simulink model "EquationsOfMotion_EOM"  (R2024b)
settings: Solver=VariableStepAuto  StartTime=0.0  StopTime=10.0  RelTol=1e-3
values from neighbouring files (symbols this model uses):
  g = 9.81    [ParameterInSI.m]    (also in start.m = 9.807)
undefined symbols (not defined in the file or in its folder): ft, INI, m, s
libraries: aerolibconvert2 x3, shared6dof x1, aerolibasang x1, aerolibanimutils x1
settings Model: Creator=the-main  LastModifiedBy=the-main

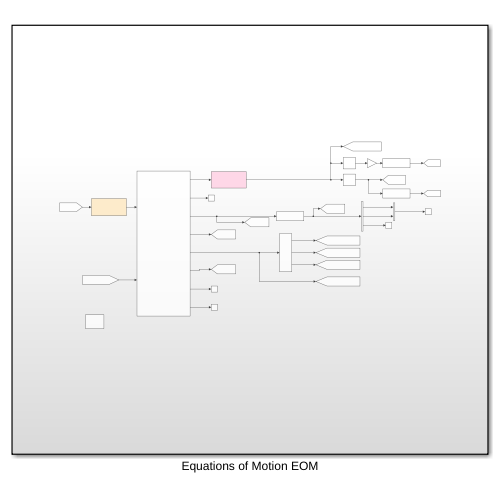
[thumbnail: Simulink's stored preview of the top-level diagram]
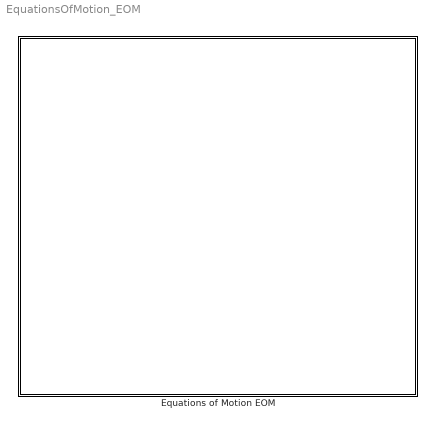
== system EquationsOfMotion_EOM ==
  Equations of Motion EOM : Subsystem

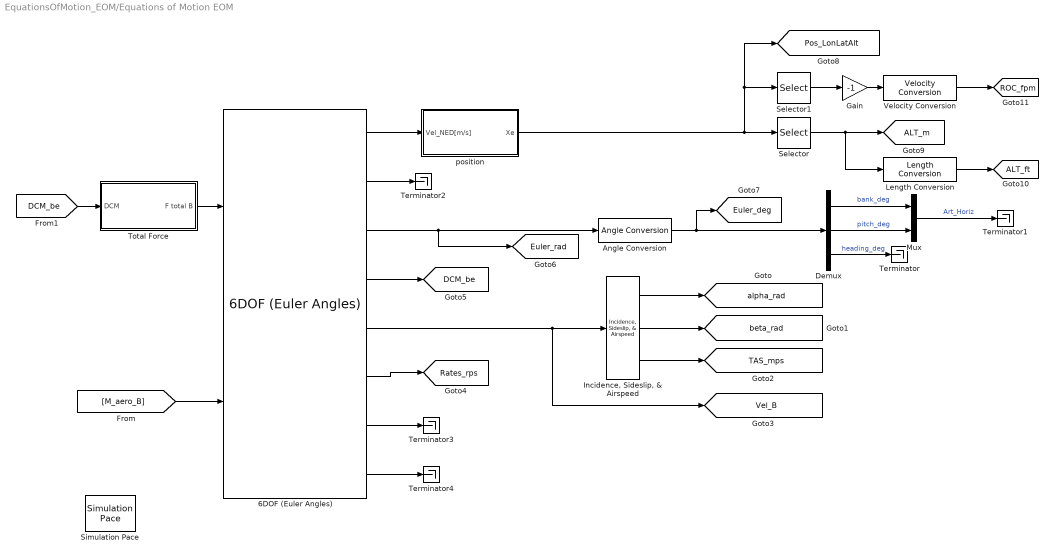
== system EquationsOfMotion_EOM/Equations of Motion EOM ==
  6DOF (Euler Angles) : shared6dof/6DOF (Euler Angles)  units=Metric (MKS)  mtype=Fixed  rep=Euler Angles  xme_0=[0 0 0]  Vm_0=[0 0 0]  eul_0=[0 0 0]  pm_0=[0 0 0]  mass_0=1.0  mass_e=0.5  mass_f=2.0  inertia=eye(3)  inertia_e=eye(3)  inertia_f=2*eye(3)  k_quat=1.0  vre_flag=on  abi_flag=off  aMode=0  xme_statename=''  Vm_statename=''  eul_statename=''  quat_statename=''  pm_statename=''  mass_statename=''
  Angle Conversion : aerolibconvert2/Angle Conversion  IU=rad  OU=deg
  Demux : Demux  Outputs=3
  Gain : Gain  Gain=-1
  "Incidence, Sideslip, & Airspeed" : aerolibasang/Incidence, Sideslip, & Airspeed
  Length Conversion : aerolibconvert2/Length Conversion  IU=m  OU=ft
  Mux : Mux  Inputs=2
  Selector : Selector  InputPortWidth=3  IndexOptions=Starting index (dialog)  Indices=3  OutputSizes=1
  Selector1 : Selector  InputPortWidth=3  IndexOptions=Starting index (dialog)  Indices=3  OutputSizes=1
  Simulation Pace : aerolibanimutils/Simulation Pace  SimulationPace=1  SleepMode=Auto  OutputPaceError=off  SampleTime=1/30
  Terminator{,1..4} (5 alike) : Terminator
  Total Force : Subsystem
  Velocity Conversion : aerolibconvert2/Velocity Conversion  IU=m/s  OU=ft/min
  position : Subsystem
  tag scope: ALT_ft=global, ALT_m=global, DCM_be=global, Euler_deg=global, Euler_rad=global, Pos_LonLatAlt=global, ROC_fpm=global, Rates_rps=global, TAS_mps=global, Vel_B=global, alpha_rad=global, beta_rad=global
  wires:
  6DOF (Euler Angles)/5 -> [Vel_B], "Incidence, Sideslip, & Airspeed"/1
  "Incidence, Sideslip, & Airspeed"/1 -> [alpha_rad]
  "Incidence, Sideslip, & Airspeed"/2 -> [beta_rad]
  "Incidence, Sideslip, & Airspeed"/3 -> [TAS_mps]
  6DOF (Euler Angles)/6 -> [Rates_rps]
  [M_aero_B] -> 6DOF (Euler Angles)/2
  Total Force/1(F total B) -> 6DOF (Euler Angles)/1
  [DCM_be] -> Total Force/1(DCM)
  6DOF (Euler Angles)/4 -> [DCM_be]
  6DOF (Euler Angles)/3 -> Angle Conversion/1, [Euler_rad]
  Angle Conversion/1 -> Demux/1, [Euler_deg]
  Demux/1 -> Mux/1  "bank_deg"
  Demux/2 -> Mux/2  "pitch_deg"
  Mux/1 -> Terminator1/1  "Art_Horiz"
  6DOF (Euler Angles)/1 -> position/1(Vel_NED[m/s])
  Demux/3 -> Terminator/1  "heading_deg"
  6DOF (Euler Angles)/2 -> Terminator2/1
  position/1(Xe) -> Selector1/1, [Pos_LonLatAlt], Selector/1
  Selector/1 -> Length Conversion/1, [ALT_m]
  Length Conversion/1 -> [ALT_ft]
  Selector1/1 -> Gain/1
  Gain/1 -> Velocity Conversion/1
  Velocity Conversion/1 -> [ROC_fpm]
  6DOF (Euler Angles)/7 -> Terminator3/1
  6DOF (Euler Angles)/8 -> Terminator4/1

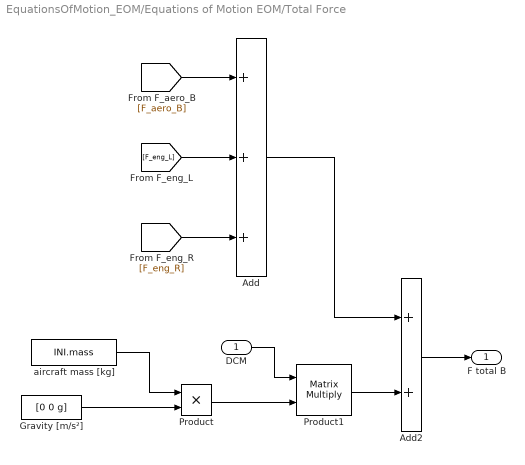
== system EquationsOfMotion_EOM/Equations of Motion EOM/Total Force ==
  DCM : Inport
  Add : Sum  Inputs=+++
  Add2 : Sum
  Gravity [m/s²] : Constant  Value=[0 0 g]
  Product : Product
  Product1 : Product  Multiplication=Matrix(*)
  aircraft mass [kg] : Constant  Value=INI.mass
  F total B : Outport  VectorParamsAs1DForOutWhenUnconnected=off
  wires:
  Add/1 -> Add2/1
  Gravity [m/s²]/1 -> Product/2
  Product1/1 -> Add2/2
  Add2/1 -> F total B/1
  Product/1 -> Product1/2
  aircraft mass [kg]/1 -> Product/1
  DCM/1 -> Product1/1
  [F_eng_R] -> Add/3
  [F_eng_L] -> Add/2
  [F_aero_B] -> Add/1

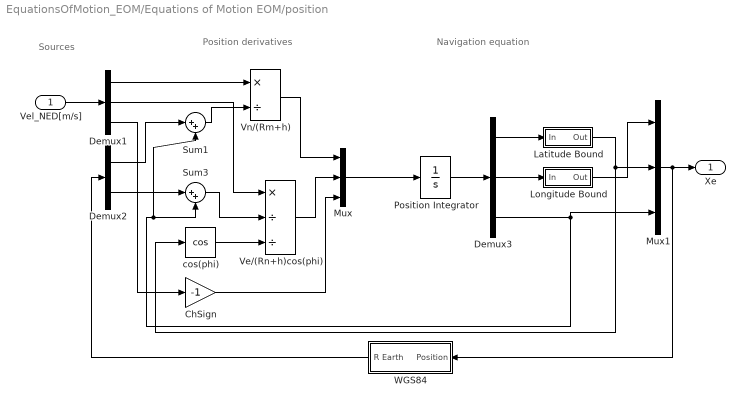
== system EquationsOfMotion_EOM/Equations of Motion EOM/position ==
  note: Navigation equation
  note: Position derivatives
  note: Sources
  Vel_NED[m/s] : Inport
  ChSign : Gain  Gain=-1  SaturateOnIntegerOverflow=on  OutDataTypeStr=Inherit: Same as input  ParamDataTypeStr=Inherit: Same as input
  Demux1 : Demux  Outputs=3
      settings: DisplayOption=none
  Demux2 : Demux  Outputs=2
      settings: DisplayOption=none
  Demux3 : Demux  Outputs=3
      settings: DisplayOption=none
  Latitude Bound : Subsystem
  Longitude Bound : Subsystem
  Mux : Mux  Inputs=3
  Mux1 : Mux  Inputs=3
  Position Integrator : Integrator  InitialCondition=INI.POS
  Sum1 : Sum  Inputs=|++
  Sum3 : Sum  Inputs=|++
  Ve/(Rn+h)cos(phi) : Product  Inputs=*//  InputSameDT=on  SaturateOnIntegerOverflow=on  OutDataTypeStr=Inherit: Same as first input
  Vn/(Rm+h) : Product  Inputs=*/  InputSameDT=on  SaturateOnIntegerOverflow=on  OutDataTypeStr=Inherit: Same as first input
  WGS84 : Subsystem
  cos(phi) : Trigonometry  Operator=cos
  Xe : Outport  VectorParamsAs1DForOutWhenUnconnected=off
  wires:
  Longitude Bound/1(Out) -> Mux1/1
  Mux1/1 -> Xe/1, WGS84/1(Position)
  cos(phi)/1 -> Ve/(Rn+h)cos(phi)/3
  Demux3/1 -> Latitude Bound/1(In)
  ChSign/1 -> Mux/3
  Latitude Bound/1(Out) -> cos(phi)/1, Mux1/2
  Vn/(Rm+h)/1 -> Mux/1
  Demux1/2 -> Ve/(Rn+h)cos(phi)/1
  Demux1/1 -> Vn/(Rm+h)/1
  Vel_NED[m/s]/1 -> Demux1/1
  Demux1/3 -> ChSign/1
  Demux3/2 -> Longitude Bound/1(In)
  Demux3/3 -> Mux1/3, Sum3/2, Sum1/2
  Ve/(Rn+h)cos(phi)/1 -> Mux/2
  WGS84/1(R Earth) -> Demux2/1
  Sum1/1 -> Vn/(Rm+h)/2
  Demux2/1 -> Sum1/1
  Demux2/2 -> Sum3/1
  Sum3/1 -> Ve/(Rn+h)cos(phi)/2
  Position Integrator/1 -> Demux3/1
  Mux/1 -> Position Integrator/1

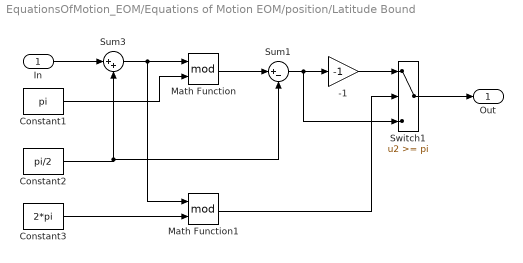
== system EquationsOfMotion_EOM/Equations of Motion EOM/position/Latitude Bound ==
  In : Inport
  -1 : Gain  Gain=-1  SaturateOnIntegerOverflow=on  OutDataTypeStr=Inherit: Same as input  ParamDataTypeStr=Inherit: Same as input
  Constant1 : Constant  Value=pi
  Constant2 : Constant  Value=pi/2
  Constant3 : Constant  Value=2*pi
  Math Function : Math  Operator=mod  SignedPower=on
  Math Function1 : Math  Operator=mod  SignedPower=on
  Sum1 : Sum  Inputs=|+-
  Sum3 : Sum  Inputs=|++
  Switch1 : Switch  Threshold=pi  SaturateOnIntegerOverflow=off  InputSameDT=off
  Out : Outport  VectorParamsAs1DForOutWhenUnconnected=off
  wires:
  -1/1 -> Switch1/1
  Switch1/1 -> Out/1
  Math Function/1 -> Sum1/1
  Sum1/1 -> Switch1/3, -1/1
  Constant3/1 -> Math Function1/2
  Constant2/1 -> Sum1/2, Sum3/2
  Constant1/1 -> Math Function/2
  In/1 -> Sum3/1
  Math Function1/1 -> Switch1/2
  Sum3/1 -> Math Function1/1, Math Function/1

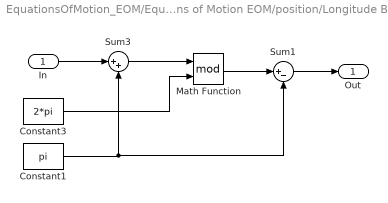
== system EquationsOfMotion_EOM/Equations of Motion EOM/position/Longitude Bound ==
  In : Inport
  Constant1 : Constant  Value=pi
  Constant3 : Constant  Value=2*pi
  Math Function : Math  Operator=mod  SignedPower=on
  Sum1 : Sum  Inputs=|+-
  Sum3 : Sum  Inputs=|++
  Out : Outport  VectorParamsAs1DForOutWhenUnconnected=off
  wires:
  Sum3/1 -> Math Function/1
  In/1 -> Sum3/1
  Constant1/1 -> Sum1/2, Sum3/2
  Constant3/1 -> Math Function/2
  Math Function/1 -> Sum1/1
  Sum1/1 -> Out/1

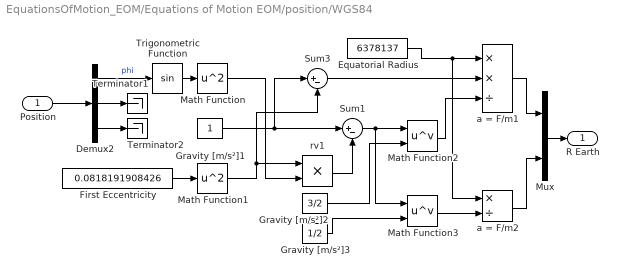
== system EquationsOfMotion_EOM/Equations of Motion EOM/position/WGS84 ==
  Position : Inport
  Demux2 : Demux  Outputs=3
  Equatorial Radius : Constant  Value=6378137
  First Eccentricity : Constant  Value=0.0818191908426
  Gravity [m/s²]1 : Constant
  Gravity [m/s²]2 : Constant  Value=3/2
  Gravity [m/s²]3 : Constant  Value=1/2
  Math Function : Math  Operator=square  SignedPower=on
  Math Function1 : Math  Operator=square  SignedPower=on
  Math Function2 : Math  Operator=pow  SignedPower=on
  Math Function3 : Math  Operator=pow  SignedPower=on
  Mux : Mux  Inputs=2
  Sum1 : Sum  Inputs=|+-
  Sum3 : Sum  Inputs=|+-
  Terminator1 : Terminator
  Terminator2 : Terminator
  Trigonometric Function : Trigonometry
  a = F/m1 : Product  Inputs=**/
  a = F/m2 : Product  Inputs=*/
  rv1 : Product
  R Earth : Outport  VectorParamsAs1DForOutWhenUnconnected=off
  wires:
  Gravity [m/s²]2/1 -> Math Function2/2
  a = F/m2/1 -> Mux/2
  Gravity [m/s²]3/1 -> Math Function3/2
  Math Function3/1 -> a = F/m2/2
  First Eccentricity/1 -> Math Function1/1
  Math Function1/1 -> Sum3/2, rv1/1
  Trigonometric Function/1 -> Math Function/1
  rv1/1 -> Sum1/2
  Sum1/1 -> Math Function3/1, Math Function2/1
  Position/1 -> Demux2/1
  Demux2/1 -> Trigonometric Function/1  "phi"
  Demux2/3 -> Terminator2/1
  Demux2/2 -> Terminator1/1
  a = F/m1/1 -> Mux/1
  Math Function/1 -> rv1/2
  Math Function2/1 -> a = F/m1/3
  Equatorial Radius/1 -> a = F/m2/1, a = F/m1/1
  Sum3/1 -> a = F/m1/2
  Gravity [m/s²]1/1 -> Sum1/1, Sum3/1
  Mux/1 -> R Earth/1
